simulink model "modelLQR"  (R2015a)
settings: Solver=ode45  StartTime=0.0  StopTime=tsim  FixedStep=1/200  RelTol=1e-3
undefined symbols (not defined in the file): A, B, Cy, D, gain, klq
settings Model: Creator=dell  LastModifiedBy=dell

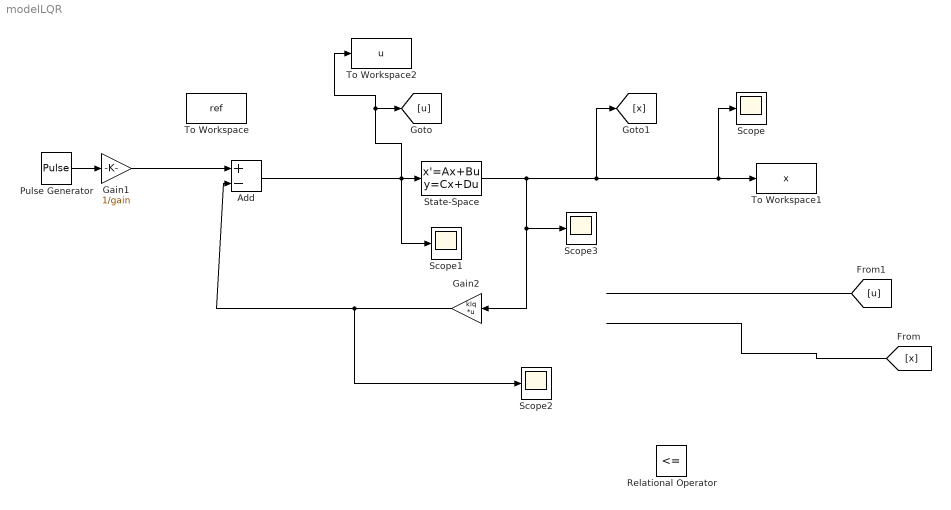
== system modelLQR ==
  Add : Sum  Inputs=+-
  Gain1 : Gain  Gain=1/gain
  Gain2 : Gain  Gain=klq  Multiplication=Matrix(K*u)
  Pulse Generator : DiscretePulseGenerator  PulseType=Time based  Period=10  PulseWidth=50  PhaseDelay=5
  Relational Operator : RelationalOperator  Operator=<=  OutDataTypeStr=boolean
  Scope{,1..3} (4 alike) : Scope
      Scope2 settings: SaveName=ScopeData2
      Scope3 settings: SaveName=ScopeData3
  State-Space : StateSpace  A=A  B=B  C=Cy  D=D  X0=0
  To Workspace : ToWorkspace  VariableName=ref  SaveFormat=Timeseries  SampleTime=1/200
  To Workspace1 : ToWorkspace  VariableName=x  SaveFormat=Timeseries  SampleTime=1/200
  To Workspace2 : ToWorkspace  VariableName=u  SaveFormat=Timeseries  SampleTime=1/200
  wires:
  Add/1 -> Scope1/1, State-Space/1, To Workspace2/1, [u]
  Pulse Generator/1 -> Gain1/1
  State-Space/1 -> Scope3/1, Gain2/1, [x], Scope/1, To Workspace1/1
  Gain1/1 -> Add/1
  [x] -> ?
  [u] -> ?
  Gain2/1 -> Scope2/1, Add/2
